simulink model "at40_pCtrl"  (R2016a)
settings: Solver=ode5  StartTime=0.0  StopTime=inf  FixedStep=0.001  RelTol=1e-3
undefined symbols (not defined in the file or in its folder): robot
libraries: dcpctrl x5, simulink x5
settings Model: SimulationMode=external  Creator=julianleland  LastModifiedBy=julianleland
settings HardwareCC: ProdBitPerLong=64  ProdLargestAtomicFloat=None  ProdHWDeviceType=Intel->x86-64  TargetBitPerLong=64  TargetBitPerPointer=64  TargetIntDivRoundTo=Zero  TargetEndianess=LittleEndian  TargetWordSize=64  TargetHWDeviceType=Intel->x86-64
settings RTWCC: SystemTargetFile=sldrt.tlc  TemplateMakefile=sldrt.tmf  Description=Simulink Desktop Real-Time  RTWCompilerOptimization=on
settings CodeAppCC: MaxIdLength=95
settings SimulinkDesktopRealTimeCC: TargetPreCompLibLocation=/Applications/MATLAB_R2016a.app/toolbox/sldrt/lib/maci64  TargetLangStandard=C89/C90 (ANSI)  SupportVariableSizeSignals=off

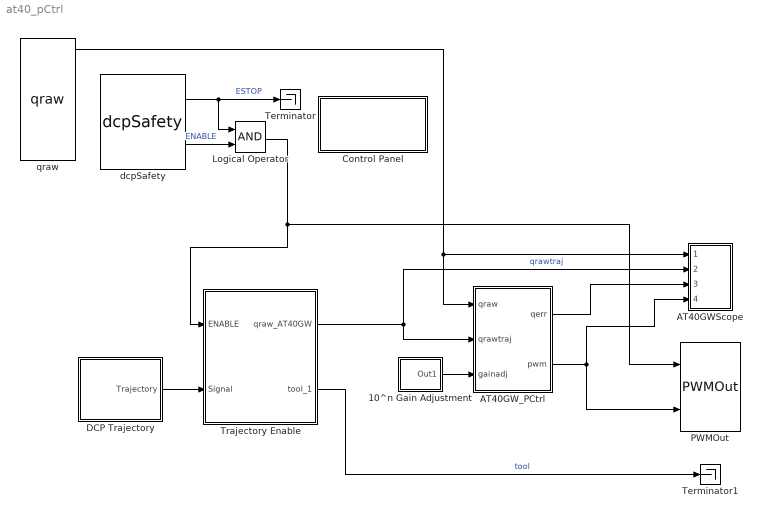
== system at40_pCtrl ==
  10^n Gain Adjustment : Subsystem
  AT40GWScope : Subsystem
  AT40GW_PCtrl : Subsystem
  Control Panel : Subsystem
  DCP Trajectory : Subsystem
  Logical Operator : Logic  AllPortsSameDT=off  OutDataTypeStr=boolean
  PWMOut : dcpctrl/PWMOut
  Terminator : Terminator
  Terminator1 : Terminator
  Trajectory Enable : Subsystem
  dcpSafety : dcpctrl/dcpSafety
  qraw : dcpctrl/qraw
  wires:
  Trajectory Enable/1(qraw_AT40GW) -> AT40GW_PCtrl/2(qrawtraj), AT40GWScope/2(Signal2)  "qrawtraj"
  AT40GW_PCtrl/2(pwm) -> PWMOut/2, AT40GWScope/4(Signal4)
  qraw/1 -> AT40GW_PCtrl/1(qraw), AT40GWScope/1(Signal1)
  AT40GW_PCtrl/1(qerr) -> AT40GWScope/3(Signal3)
  10^n Gain Adjustment/1(Out1) -> AT40GW_PCtrl/3("gainadj ")
  Logical Operator/1 -> Trajectory Enable/1(ENABLE), PWMOut/1
  dcpSafety/1 -> Logical Operator/1, Terminator/1  "ESTOP"
  dcpSafety/2 -> Logical Operator/2  "ENABLE"
  DCP Trajectory/1(Trajectory) -> Trajectory Enable/2(Signal)
  Trajectory Enable/2(tool_1) -> Terminator1/1  "tool"

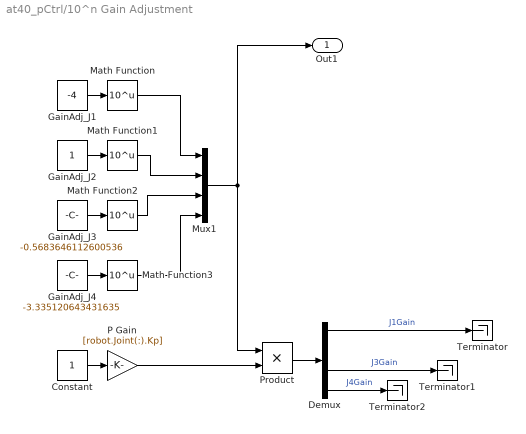
== system at40_pCtrl/10^n Gain Adjustment ==
  Constant : Constant
  Demux : Demux
  GainAdj_J1 : Constant  Value=-4
  GainAdj_J2 : Constant
  GainAdj_J3 : Constant  Value=-0.5683646112600536
  GainAdj_J4 : Constant  Value=-3.335120643431635
  Math Function{,1..3} (4 alike) : Math  Operator=10^u  SaturateOnIntegerOverflow=on
  Mux1 : Mux
  P Gain : Gain  Gain=[robot.Joint(:).Kp]
  Product : Product
  Terminator : Terminator
  Terminator1 : Terminator
  Terminator2 : Terminator
  Out1 : Outport
  wires:
  Math Function1/1 -> Mux1/2
  Math Function/1 -> Mux1/1
  Mux1/1 -> Out1/1, Product/1
  Math Function3/1 -> Mux1/4
  Math Function2/1 -> Mux1/3
  GainAdj_J1/1 -> Math Function/1
  GainAdj_J2/1 -> Math Function1/1
  GainAdj_J3/1 -> Math Function2/1
  GainAdj_J4/1 -> Math Function3/1
  Constant/1 -> P Gain/1
  P Gain/1 -> Product/2
  Product/1 -> Demux/1
  Demux/4 -> Terminator2/1  "J4Gain"
  Demux/1 -> Terminator/1  "J1Gain"
  Demux/3 -> Terminator1/1  "J3Gain"

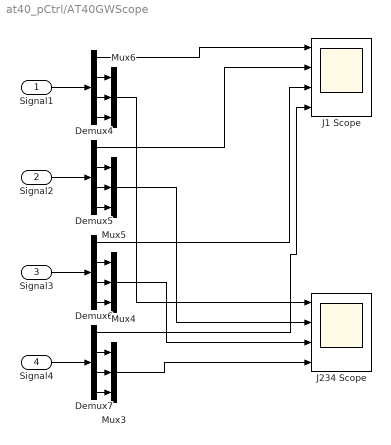
== system at40_pCtrl/AT40GWScope ==
  Signal1 : Inport
  Signal2 : Inport  Port=2
  Signal3 : Inport  Port=3
  Signal4 : Inport  Port=4
  Demux{4..7} (4 alike) : Demux
  J1 Scope : Scope  NumInputPorts=4
  J234 Scope : Scope  NumInputPorts=4
  Mux{3..6} (4 alike) : Mux  Inputs=3
  wires:
  Demux7/1 -> J1 Scope/4
  Demux6/1 -> J1 Scope/3
  Demux5/1 -> J1 Scope/2
  Demux4/1 -> J1 Scope/1
  Mux3/1 -> J234 Scope/4
  Demux7/3 -> Mux3/2
  Demux7/4 -> Mux3/3
  Demux6/3 -> Mux4/2
  Demux7/2 -> Mux3/1
  Demux6/2 -> Mux4/1
  Demux6/4 -> Mux4/3
  Mux4/1 -> J234 Scope/3
  Demux5/2 -> Mux5/1
  Demux5/3 -> Mux5/2
  Demux5/4 -> Mux5/3
  Mux5/1 -> J234 Scope/2
  Mux6/1 -> J234 Scope/1
  Demux4/2 -> Mux6/1
  Demux4/4 -> Mux6/3
  Demux4/3 -> Mux6/2
  Signal1/1 -> Demux4/1
  Signal2/1 -> Demux5/1
  Signal3/1 -> Demux6/1
  Signal4/1 -> Demux7/1

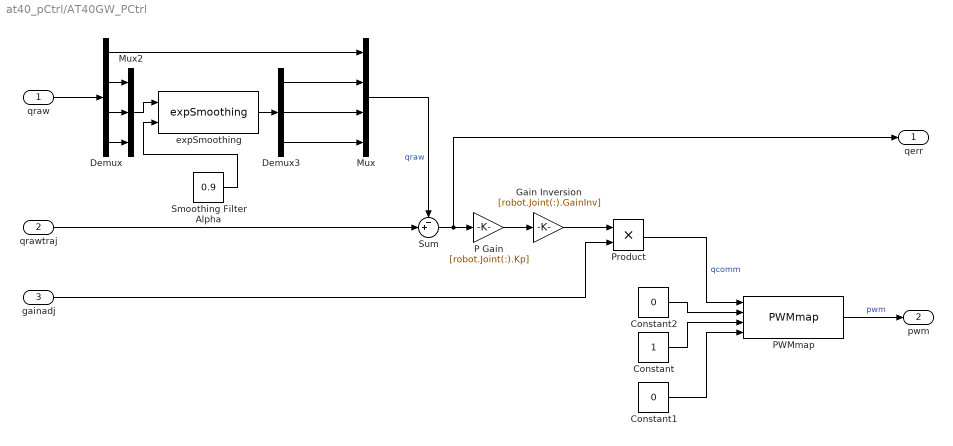
== system at40_pCtrl/AT40GW_PCtrl ==
  qraw : Inport
  qrawtraj : Inport  Port=2
  "gainadj " : Inport  Port=3
  Constant : Constant
  Constant1 : Constant  Value=0
  Constant2 : Constant  Value=0
  Demux : Demux
  Demux3 : Demux  Outputs=3
  Gain Inversion : Gain  Gain=[robot.Joint(:).GainInv]
  Mux : Mux
  Mux2 : Mux  Inputs=3
  P Gain : Gain  Gain=[robot.Joint(:).Kp]
  PWMmap : dcpctrl/PWMmap
  Product : Product
  Smoothing Filter Alpha : Constant  Value=0.9
  Sum : Sum  Inputs=-+|
  expSmoothing : dcpctrl/expSmoothing
  qerr : Outport
  pwm : Outport  Port=2
  wires:
  qrawtraj/1 -> Sum/2
  Mux/1 -> Sum/1  "qraw"
  Demux/1 -> Mux/1
  expSmoothing/1 -> Demux3/1
  Demux3/2 -> Mux/3
  Demux3/1 -> Mux/2
  Demux3/3 -> Mux/4
  Smoothing Filter Alpha/1 -> expSmoothing/2
  Mux2/1 -> expSmoothing/1
  Sum/1 -> qerr/1, P Gain/1
  PWMmap/1 -> pwm/1  "pwm"
  Product/1 -> PWMmap/1  "qcomm"
  P Gain/1 -> Gain Inversion/1
  "gainadj "/1 -> Product/2
  Gain Inversion/1 -> Product/1
  Constant/1 -> PWMmap/3
  Constant1/1 -> PWMmap/4
  Constant2/1 -> PWMmap/2
  Demux/4 -> Mux2/3
  Demux/3 -> Mux2/2
  Demux/2 -> Mux2/1
  qraw/1 -> Demux/1

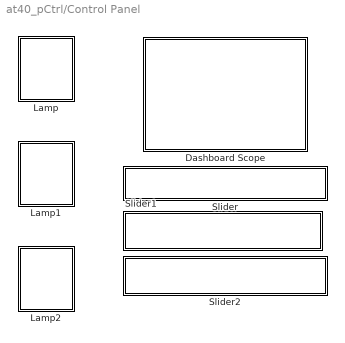
== system at40_pCtrl/Control Panel ==
  Dashboard Scope : Subsystem  DialogController=hmiCreateDDGDialog  IsWebBlock=on  mask(MWDashboardBlock){webBlockId=c47a9cdb-cb75-452f-8799-f21a48509ad2, webBlockType=sdiscope, ShowInitialText=on, HMISrcModelName=at40_pCtrl}
      mask prompts: webBlockId "WebBlock Id"; webBlockType "WebBlock Type"; HMISrcModelName "Source Model"
      mask Help: helpview([docroot '/mapfiles/simulink.map'], 'hmi_scope')
      mask Display:
      | if strcmp(get_param(bdroot(gcb),'BlockDiagramType'), 'library')
      |     image([(matlabroot) '/toolbox/simulink/hmi/icons/DashboardScope.png']);
      | end
  Lamp : Subsystem  DialogController=hmiCreateDDGDialog  IsWebBlock=on  mask(MWDashboardBlock){webBlockId=ed38c6ac-d807-4a86-a2c0-97ede734ce07, webBlockType=lamp, ShowInLibBrowser=on, ShowInitialText=on, HMISrcModelName=at40_pCtrl}
      mask prompts: webBlockType "WebBlock Type"; HMISrcModelName "Source Model"
      mask Help: helpview([docroot '/mapfiles/simulink.map'], 'hmi_lamp')
      mask Display:
      | if strcmp(get_param(bdroot(gcb),'BlockDiagramType'), 'library')
      |     image([(matlabroot) '/toolbox/simulink/hmi/icons/Lamp.png']);
      | end
  Lamp1 : Subsystem  DialogController=hmiCreateDDGDialog  IsWebBlock=on  mask(MWDashboardBlock){webBlockId=7d773b0c-0afc-40d6-90a6-84b2767f4ba1, webBlockType=lamp, ShowInLibBrowser=on, ShowInitialText=on, HMISrcModelName=at40_pCtrl}
      mask prompts: webBlockType "WebBlock Type"; HMISrcModelName "Source Model"
      mask Help: helpview([docroot '/mapfiles/simulink.map'], 'hmi_lamp')
      mask Display:
      | if strcmp(get_param(bdroot(gcb),'BlockDiagramType'), 'library')
      |     image([(matlabroot) '/toolbox/simulink/hmi/icons/Lamp.png']);
      | end
  Lamp2 : Subsystem  DialogController=hmiCreateDDGDialog  IsWebBlock=on  mask(MWDashboardBlock){webBlockId=76a982f2-5229-4926-b658-81f142de1416, webBlockType=lamp, ShowInLibBrowser=on, ShowInitialText=on, HMISrcModelName=at40_pCtrl}
      mask prompts: webBlockType "WebBlock Type"; HMISrcModelName "Source Model"
      mask Help: helpview([docroot '/mapfiles/simulink.map'], 'hmi_lamp')
      mask Display:
      | if strcmp(get_param(bdroot(gcb),'BlockDiagramType'), 'library')
      |     image([(matlabroot) '/toolbox/simulink/hmi/icons/Lamp.png']);
      | end
  Slider : Subsystem  DialogController=hmiCreateDDGDialog  IsWebBlock=on  mask(MWDashboardBlock){webBlockId=1e5f77f3-b054-4aef-b3b7-666c2ac5e1ba, webBlockType=slider, ShowInLibBrowser=on, ShowInitialText=on, HMISrcModelName=at40_pCtrl}
      mask prompts: webBlockId "WebBlock Id"; webBlockType "WebBlock Type"; HMISrcModelName "Source Model"
      mask Help: helpview([docroot '/mapfiles/simulink.map'], 'hmi_slider')
      mask Display:
      | if strcmp(get_param(bdroot(gcb),'BlockDiagramType'), 'library')
      |     image([(matlabroot) '/toolbox/simulink/hmi/icons/Slider.png']);
      | end
  Slider1 : Subsystem  DialogController=hmiCreateDDGDialog  IsWebBlock=on  mask(MWDashboardBlock){webBlockId=acd0711e-5899-49c7-8654-ee1ca4e90d52, webBlockType=slider, ShowInLibBrowser=on, ShowInitialText=on, HMISrcModelName=at40_pCtrl}
      mask prompts: webBlockId "WebBlock Id"; webBlockType "WebBlock Type"; HMISrcModelName "Source Model"
      mask Help: helpview([docroot '/mapfiles/simulink.map'], 'hmi_slider')
      mask Display:
      | if strcmp(get_param(bdroot(gcb),'BlockDiagramType'), 'library')
      |     image([(matlabroot) '/toolbox/simulink/hmi/icons/Slider.png']);
      | end
  Slider2 : Subsystem  DialogController=hmiCreateDDGDialog  IsWebBlock=on  mask(MWDashboardBlock){webBlockId=c727be91-e8d7-4734-bda2-adb83f8e324c, webBlockType=slider, ShowInLibBrowser=on, ShowInitialText=on, HMISrcModelName=at40_pCtrl}
      mask prompts: webBlockId "WebBlock Id"; webBlockType "WebBlock Type"; HMISrcModelName "Source Model"
      mask Help: helpview([docroot '/mapfiles/simulink.map'], 'hmi_slider')
      mask Display:
      | if strcmp(get_param(bdroot(gcb),'BlockDiagramType'), 'library')
      |     image([(matlabroot) '/toolbox/simulink/hmi/icons/Slider.png']);
      | end

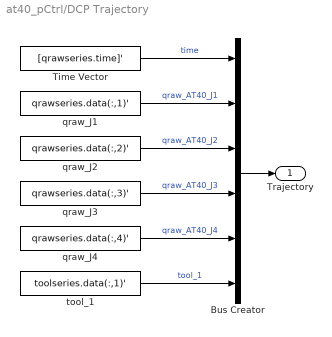
== system at40_pCtrl/DCP Trajectory ==
  Bus Creator : BusCreator  Inputs='time','qraw_AT40_J1','qraw_AT40_J2','qraw_AT40_J3','qraw_AT40_J4','tool_1'
  Time Vector : FromWorkspace  VariableName=[qrawseries.time]'  SampleTime=0
  qraw_J1 : FromWorkspace  VariableName=qrawseries.data(:,1)'  SampleTime=0
  qraw_J2 : FromWorkspace  VariableName=qrawseries.data(:,2)'  SampleTime=0
  qraw_J3 : FromWorkspace  VariableName=qrawseries.data(:,3)'  SampleTime=0
  qraw_J4 : FromWorkspace  VariableName=qrawseries.data(:,4)'  SampleTime=0
  tool_1 : FromWorkspace  VariableName=toolseries.data(:,1)'  SampleTime=0
  Trajectory : Outport
  wires:
  tool_1/1 -> Bus Creator/6  "tool_1"
  Bus Creator/1 -> Trajectory/1
  qraw_J4/1 -> Bus Creator/5  "qraw_AT40_J4"
  qraw_J2/1 -> Bus Creator/3  "qraw_AT40_J2"
  Time Vector/1 -> Bus Creator/1  "time"
  qraw_J3/1 -> Bus Creator/4  "qraw_AT40_J3"
  qraw_J1/1 -> Bus Creator/2  "qraw_AT40_J1"

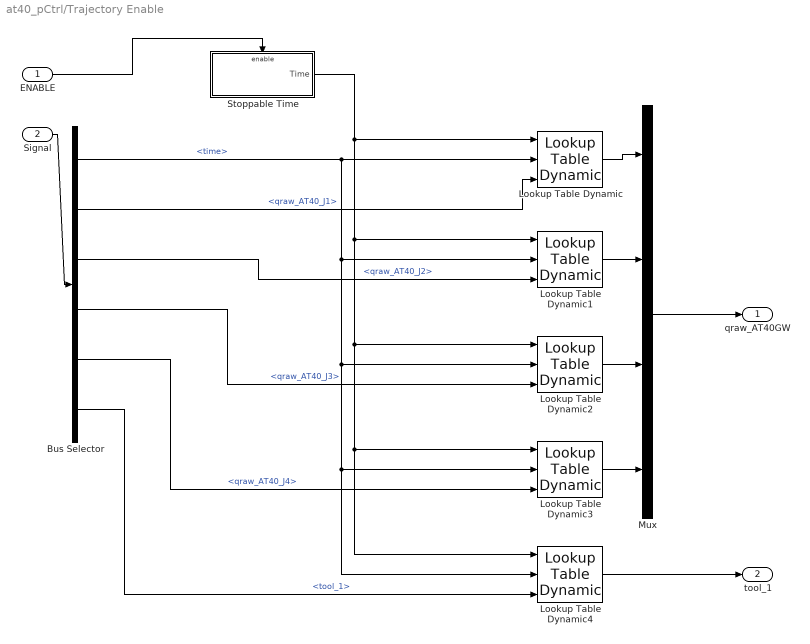
== system at40_pCtrl/Trajectory Enable ==
  ENABLE : Inport
  Signal : Inport  Port=2
  Bus Selector : BusSelector  OutputSignals=time,qraw_AT40_J1,qraw_AT40_J2,qraw_AT40_J3,qraw_AT40_J4,tool_1
  Lookup Table Dynamic{,1..4} (5 alike) : simulink/Lookup Tables/Lookup Table Dynamic  LookUpMeth=Interpolation-Use End Values  OutDataTypeStr=Inherit: Inherit via back propagation  OutDataType=fixdt('double')  OutScaling=2^-10  DoSatur=off
  Mux : Mux
  Stoppable Time : Subsystem  TreatAsAtomicUnit=on
  qraw_AT40GW : Outport
  tool_1 : Outport  Port=2
  wires:
  ENABLE/1 -> Stoppable Time/Enable
  Stoppable Time/1(Time) -> Lookup Table Dynamic4/1, Lookup Table Dynamic3/1, Lookup Table Dynamic2/1, Lookup Table Dynamic1/1, Lookup Table Dynamic/1
  Bus Selector/5 -> Lookup Table Dynamic3/3  "<qraw_AT40_J4>"
  Lookup Table Dynamic/1 -> Mux/1
  Bus Selector/2 -> Lookup Table Dynamic/3  "<qraw_AT40_J1>"
  Bus Selector/3 -> Lookup Table Dynamic1/3  "<qraw_AT40_J2>"
  Bus Selector/1 -> Lookup Table Dynamic4/2, Lookup Table Dynamic3/2, Lookup Table Dynamic2/2, Lookup Table Dynamic1/2, Lookup Table Dynamic/2  "<time>"
  Bus Selector/4 -> Lookup Table Dynamic2/3  "<qraw_AT40_J3>"
  Lookup Table Dynamic3/1 -> Mux/4
  Lookup Table Dynamic2/1 -> Mux/3
  Lookup Table Dynamic1/1 -> Mux/2
  Mux/1 -> qraw_AT40GW/1
  Signal/1 -> Bus Selector/1
  Lookup Table Dynamic4/1 -> tool_1/1
  Bus Selector/6 -> Lookup Table Dynamic4/3  "<tool_1>"

== system at40_pCtrl/Control Panel/Dashboard Scope ==

== system at40_pCtrl/Control Panel/Lamp ==

== system at40_pCtrl/Control Panel/Lamp1 ==

== system at40_pCtrl/Control Panel/Lamp2 ==

== system at40_pCtrl/Control Panel/Slider ==

== system at40_pCtrl/Control Panel/Slider1 ==

== system at40_pCtrl/Control Panel/Slider2 ==

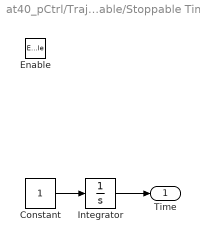
== system at40_pCtrl/Trajectory Enable/Stoppable Time ==
  Enable : EnablePort
  Constant : Constant
  Integrator : Integrator
  Time : Outport
  wires:
  Constant/1 -> Integrator/1
  Integrator/1 -> Time/1
